simulink library "check_valve"  (R2023b)
settings: Solver=VariableStepAuto  StartTime=0.0  StopTime=10.0  RelTol=1e-3
libraries: FAM_quasi_static_outflow x1
settings Model: Creator=cmmcguir  LastModifiedBy=Carson

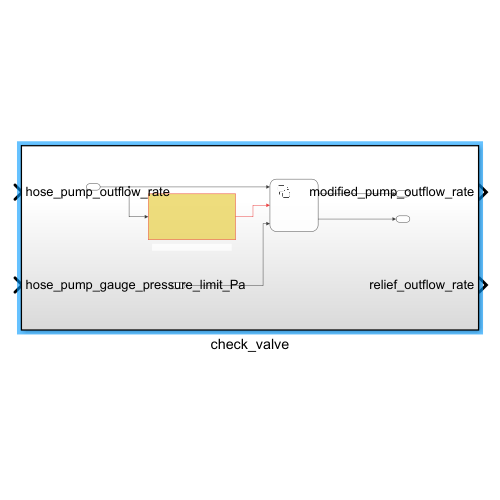
[thumbnail: Simulink's stored preview of the top-level diagram]
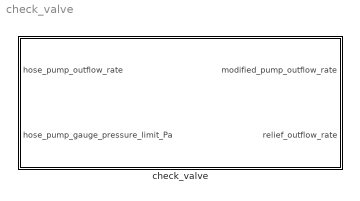
== system check_valve ==
  check_valve : Subsystem

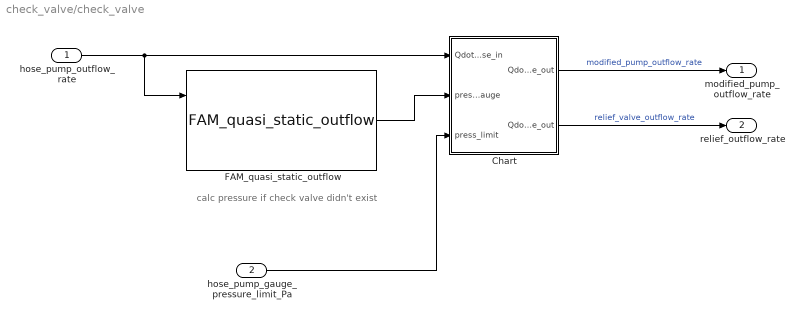
== system check_valve/check_valve ==
  note: calc pressure if check valve didn't exist
  hose_pump_outflow_rate : Inport
  hose_pump_gauge_pressure_limit_Pa : Inport  Port=2
  Chart : Stateflow chart  TreatAsAtomicUnit=on
  FAM_quasi_static_outflow : FAM_quasi_static_outflow/FAM_quasi_static_outflow  SystemSampleTime=-1  VariantActivationTime=update diagram  AllowFlexibleInterface=on  Latency=0  AutoFrameSizeCalculation=off
  modified_pump_outflow_rate : Outport
  relief_outflow_rate : Outport  Port=2
  wires:
  hose_pump_gauge_pressure_limit_Pa/1 -> Chart/3(press_limit)
  hose_pump_outflow_rate/1 -> FAM_quasi_static_outflow/1, Chart/1(Qdot_hose_in)
  Chart/1(Qdot_hose_out) -> modified_pump_outflow_rate/1  "modified_pump_outflow_rate"
  Chart/2(Qdot_valve_out) -> relief_outflow_rate/1  "relief_valve_outflow_rate"
  FAM_quasi_static_outflow/1 -> Chart/2(press_gauge)

== stateflow chart check_valve/Chart ==
  state below_lim
    en, du:
    Qdot_hose_out = Qdot_hose_in;
    Qdot_valve_out = 0;
  state above_lim
    en, du:
    Qdot_valve_out = max([0, Qdot_hose_in - Qdot_hose_out]);
  (default) -> below_lim
  below_lim -> above_lim : [press_gauge > press_limit]
  above_lim -> below_lim : [press_gauge <= press_limit]
  data: Qdot_hose_in input; press_gauge input; press_limit input; Qdot_hose_out output; Qdot_valve_out output
